simulink model "Force_and_Torque"  (R2018a)
settings: Solver=VariableStepAuto  StartTime=0.0  StopTime=10.0  RelTol=1e-3
model workspace (MAT data in the model file):
  k = Simulink.Parameter
  k.DataType = 'auto'
  k.Dimensions = [0 0]
settings Model: Creator=Ibrahim  LastModifiedBy=Ibrahim

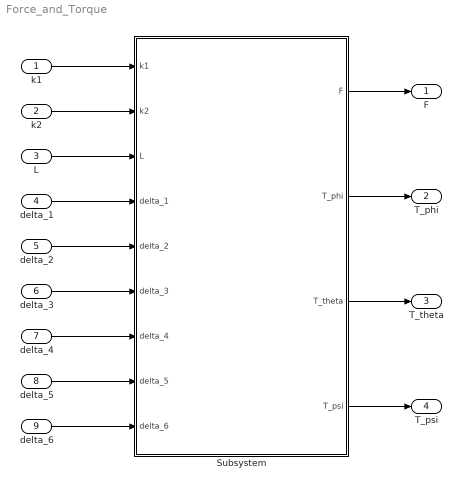
== system Force_and_Torque ==
  k1 : Inport
  k2 : Inport  Port=2
  L : Inport  Port=3
  delta_1 : Inport  Port=4
  delta_2 : Inport  Port=5
  delta_3 : Inport  Port=6
  delta_4 : Inport  Port=7
  delta_5 : Inport  Port=8
  delta_6 : Inport  Port=9
  Subsystem : Subsystem
  F : Outport
  T_phi : Outport  Port=2
  T_theta : Outport  Port=3
  T_psi : Outport  Port=4
  wires:
  k1/1 -> Subsystem/1(k1)
  k2/1 -> Subsystem/2(k2)
  L/1 -> Subsystem/3(L)
  delta_1/1 -> Subsystem/4(delta_1)
  delta_2/1 -> Subsystem/5(delta_2)
  delta_3/1 -> Subsystem/6(delta_3)
  delta_4/1 -> Subsystem/7(delta_4)
  delta_5/1 -> Subsystem/8(delta_5)
  delta_6/1 -> Subsystem/9(delta_6)
  Subsystem/1(F) -> F/1
  Subsystem/2(T_phi) -> T_phi/1
  Subsystem/3(T_theta) -> T_theta/1
  Subsystem/4(T_psi) -> T_psi/1

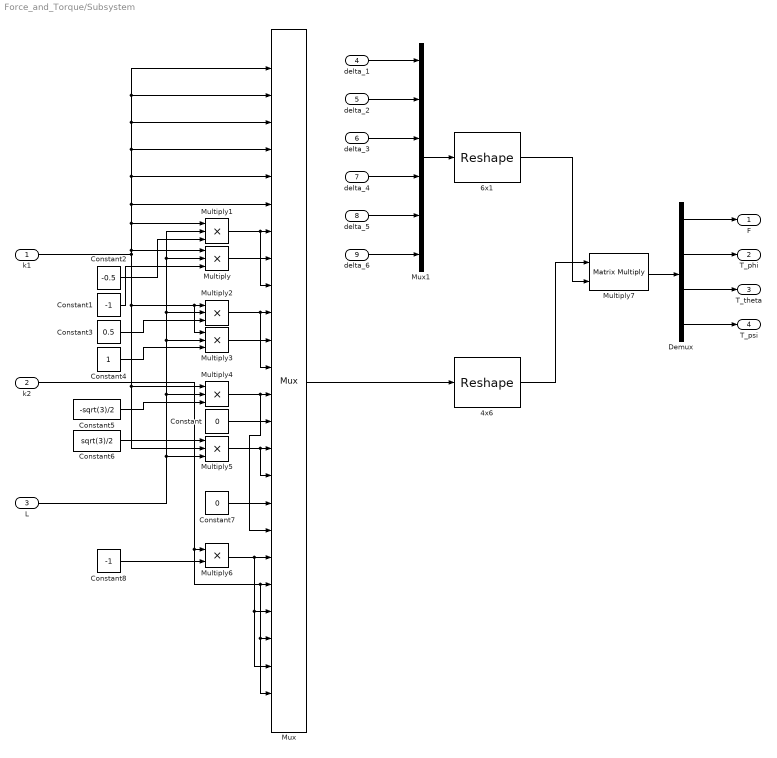
== system Force_and_Torque/Subsystem ==
  k1 : Inport
  k2 : Inport  Port=2
  L : Inport  Port=3
  delta_1 : Inport  Port=4
  delta_2 : Inport  Port=5
  delta_3 : Inport  Port=6
  delta_4 : Inport  Port=7
  delta_5 : Inport  Port=8
  delta_6 : Inport  Port=9
  4x6 : Reshape  OutputDimensionality=Customize  OutputDimensions=[4,6]
  6x1 : Reshape  OutputDimensionality=Customize  OutputDimensions=[6,1]
  Constant : Constant  Value=0  VectorParams1D=off
  Constant1 : Constant  Value=-1  VectorParams1D=off
  Constant2 : Constant  Value=-0.5  VectorParams1D=off
  Constant3 : Constant  Value=0.5  VectorParams1D=off
  Constant4 : Constant  VectorParams1D=off
  Constant5 : Constant  Value=-sqrt(3)/2  VectorParams1D=off
  Constant6 : Constant  Value=sqrt(3)/2  VectorParams1D=off
  Constant7 : Constant  Value=0  VectorParams1D=off
  Constant8 : Constant  Value=-1  VectorParams1D=off
  Demux : Demux
  Multiply{,1..5} (6 alike) : Product  Inputs=3
  Multiply6 : Product
  Multiply7 : Product  Multiplication=Matrix(*)
  Mux : Mux  Inputs=24
      settings: DisplayOption=signals
  Mux1 : Mux  Inputs=6
  F : Outport
  T_phi : Outport  Port=2
  T_theta : Outport  Port=3
  T_psi : Outport  Port=4
  wires:
  Demux/3 -> T_theta/1
  Constant3/1 -> Multiply2/3
  k1/1 -> Multiply5/2, Multiply4/1, Multiply3/1, Multiply2/1, Multiply1/1, Mux/6, Mux/5, Mux/4, Mux/3, Mux/2, Mux/1, Multiply/1
  Multiply6/1 -> Mux/21, Mux/23, Mux/19
  L/1 -> Multiply5/3, Multiply4/2, Multiply3/2, Multiply2/2, Multiply1/2, Multiply/2
  Constant6/1 -> Multiply5/1
  Multiply1/1 -> Mux/9, Mux/7
  Mux/1 -> 4x6/1
  Multiply2/1 -> Mux/12, Mux/10
  Constant7/1 -> Mux/17
  delta_6/1 -> Mux1/6
  k2/1 -> Mux/22, Mux/24, Mux/20, Multiply6/1
  Multiply3/1 -> Mux/11
  Constant4/1 -> Multiply3/3
  Multiply4/1 -> Mux/18, Mux/13
  Multiply5/1 -> Mux/16, Mux/15
  delta_1/1 -> Mux1/1
  Constant1/1 -> Multiply/3
  delta_2/1 -> Mux1/2
  delta_3/1 -> Mux1/3
  Constant8/1 -> Multiply6/2
  delta_5/1 -> Mux1/5
  Demux/1 -> F/1
  Multiply/1 -> Mux/8
  Constant2/1 -> Multiply1/3
  Constant/1 -> Mux/14
  delta_4/1 -> Mux1/4
  Demux/2 -> T_phi/1
  Mux1/1 -> 6x1/1
  Constant5/1 -> Multiply4/3
  Demux/4 -> T_psi/1
  4x6/1 -> Multiply7/1
  6x1/1 -> Multiply7/2
  Multiply7/1 -> Demux/1
